simulink model "tqdtqr_rebuild_V3"  (R2021b)
settings: Solver=VariableStepAuto  StartTime=0.0  StopTime=10.0  RelTol=1e-3
undefined symbols (not defined in the file): ATQD_AfterTqMinGain_X_Deg, ATQD_APSCreepBaseTqD_X_kph, ATQD_APSCreepBaseTqD_Y_Deg, ATQD_APSCreepBaseTqR_X_kph, ATQD_APSCreepBaseTqR_Y_Deg, ATQD_APSCreepIterm_X_kph, ATQD_APSCreepIterm_Y_kph, ATQD_APSCreepPterm_X_kph, ATQD_APSCreepPterm_Y_kph, ATQD_APSDecReq_X_kph, ATQD_APSDecReq_Y_mps2, ATQD_APSDecReqCMD_X_kph, ATQD_APSDecReqTs_X_pct, ATQD_APSDecTimeGain_X_Deg, ATQD_APSDecTimeGain_Y_s, ATQD_APSReqLowSpd_X_Deg, ATQD_AutoHoldReleaseBPS_X_Deg, ATQD_AWDLoadTrqnsGain_X_kg, ATQD_AWDLoadTrqnsGain_Y_pct, ATQD_BOSEnBPSPosn_X_kph, ATQD_BOSMap_X_rpm, ATQD_BOSMap_Y_pct, ATQD_CreepBaseTqD_X_kph, ATQD_CreepBaseTqD_Y_Deg, ATQD_CreepBaseTqR_X_kph, ATQD_CreepBaseTqR_Y_Deg, ATQD_CreepBPSDisPosn_X_Deg, ATQD_CreepBPSDisPosnR_X_Deg, ATQD_CreepBPSEnPosn_X_Deg, ATQD_CreepBPSEnPosnR_X_Deg, ATQD_CreepDeltaTq_X_kph, ATQD_CreepIterm_X_kph, ATQD_CreepIterm_Y_kph, ATQD_CreepItermMaxLimit_X_pct, ATQD_CreepPreloadTime_X_kph, ATQD_CreepPreloadTq_X_kph, ATQD_CreepPreloadTq_Y_s, ATQD_CreepProtTq_X_Deg, ATQD_CreepPterm_X_kph, ATQD_CreepPterm_Y_kph, ATQD_CreepRrTqSpRat_X_rpm, ATQD_CreepRrTqSpRat_Y_Nm, ATQD_CreepTargetSpdD_X_pct, ATQD_CreepTargetSpdR_X_pct, ATQD_CreepUpLimitTq_X_rpm, ATQD_DecIneOPDHoldEnDelay_X_Deg, ATQD_DecIneOPDHoldEnDelay_Y_bar, ATQD_ECOTqMapD_X_rpm, ATQD_ECOTqMapD_Y_pct, ATQD_EMTqMapD_X_rpm, ATQD_EMTqMapD_Y_pct, ATQD_EOPDTqMapDCon_X_rpm, ATQD_EOPDTqMapDCon_Y_Deg, ATQD_EstInitVehWeight_X_c, ATQD_FAfterTqCMDGain_X_rpm, ATQD_FAfterTqCMDGain_Y_pct, ATQD_ForceLowSpd_X_Deg, ATQD_ForcePLimitSpd_X_Deg, ATQD_FrLossMAPLowV_X_rpm, ATQD_FrLossMAPLowV_Y_Nm ... (+949)
libraries: simulink x235, hcu_lib x208, tqr x63, tqd x6
(part 30 of 37)

== system tqdtqr_rebuild_V3/Input_Convert/Signal function/SWC1 SWC2 status/SWC2_Subsystem/Speed Setting Mode/ACC Speed Setting ON ==
  note: ACC limit speed setting
  note: ACCSetSpd_241018
  VTQD_SWC2ScrollUpSta_enum : Inport
  VTQD_SWC2ScrollDownSta_enum : Inport  Port=2
  VVMC_LVDAACCStatusInformation_flg : Inport  Port=3
  VTQD_SpdLim4SetSpd_raw32 : Inport  Port=4
  VINP_ADASACCSta_enum : Inport  Port=5
  VINP_Distanceunit_flg : Inport  Port=6
  VINP_SmartEcoModeSW_flg : Inport  Port=7
  VINP_IVIACCAdaptiveSta_flg : Inport  Port=8
  VTQD_Set2MeterSpd_flg : Inport  Port=9
  VTQD_SetRoadSpdLim_flg : Inport  Port=10
  VINP_ADASSLIFSpdLim_enum : Inport  Port=11
  VTQD_LScrollPressShort_flg : Inport  Port=12
  VVMC_MeterIndSpeed_raw32 : Inport  Port=13
  VTQD_SWC2ScrollDownSta_flg : Inport  Port=14
  VTQD_SWC2ScrollUpSta_flg : Inport  Port=15
  VTQD_LastSetSpd_kph : Inport  Port=16
  Action Port : ActionPort  InitializeStates=reset  ActionPortLabel=if(u1 ~= 0)
  " 20" : Constant  Value=KTQD_ACCActiveMetSpdLoMPH_mph
  " 30kph" : Constant  Value=KTQD_ACCActiveMetSpdLo_kph
  105 : Constant  Value=KTQD_ACCActiveMetSpdHiMPH_mph
  180kph : Constant  Value=KTQD_ACCActiveMetSpdHi_kph
  2 : Constant  Value=KTQD_SmartEcoLimitSpd_kph
  3 : Constant  Value=KTQD_SmartEcoLimitSpd_mph
  5 : Constant  Value=KTQD_SetSpdDeltaLongMPH_mph
  5kph : Constant  Value=KTQD_SetSpdDeltaLong_kph
  ACCSetSpd_2506 : Stateflow chart  TreatAsAtomicUnit=on
  AND1 : Logic  AllPortsSameDT=off  OutDataTypeStr=boolean
  Cast To Single : DataTypeConversion  OutDataTypeStr=int8
  Constant126 : Constant  Value=0x0  OutDataTypeStr=uint8
  Equal53 : RelationalOperator  Operator=~=  OutDataTypeStr=boolean  RndMeth=Simplest
  ONE : Constant  Value=ONE_INT
  Relational Operator2 : RelationalOperator  Operator===  OutDataTypeStr=boolean  RndMeth=Simplest
  Relational Operator4 : RelationalOperator  Operator===  OutDataTypeStr=boolean  RndMeth=Simplest
  Round : Rounding  Operator=round
  Switch{1..6} (6 alike) : Switch  Criteria=u2 ~= 0
      settings: AttributesFormatString=%<Criteria>
  standby : Constant  Value=ENUM_ADASACCSTA_STANDBY
  zero : Constant  Value=ZERO_INT
  VTQD_ACCSetSpd_kph : Outport
  wires:
  [VTQD_LastSetSpd_kph] -> ACCSetSpd_2506/18(VTQD_LastSetSpd_kph)
  VTQD_LastSetSpd_kph/1 -> [VTQD_LastSetSpd_kph]
  VTQD_SWC2ScrollUpSta_flg/1 -> [VTQD_SWC2ScrollUpSta_flg]
  VTQD_SWC2ScrollDownSta_flg/1 -> [VTQD_SWC2ScrollDownSta_flg]
  [VTQD_SWC2ScrollDownSta_flg] -> ACCSetSpd_2506/17(VTQD_SWC2ScrollDownSta_flg)
  [VTQD_SWC2ScrollUpSta_flg] -> ACCSetSpd_2506/16(VTQD_SWC2ScrollUpSta_flg)
  [VTQD_ADASSLIFSpdLimDet_flg] -> ACCSetSpd_2506/12(VTQD_ADASSLIFSpdLimDet_flg)
  Equal53/1 -> [VTQD_ADASSLIFSpdLimDet_flg]  "VTQD_ADASSLIFSpdLimDet_flg"
  [VVMC_MeterIndSpeed_raw32] -> ACCSetSpd_2506/15(VVMC_MeterIndSpeed_raw32)
  VVMC_MeterIndSpeed_raw32/1 -> [VVMC_MeterIndSpeed_raw32]
  [VTQD_LScrollPressShort_flg] -> ACCSetSpd_2506/13(VTQD_LScrollPressShort_flg)
  VTQD_LScrollPressShort_flg/1 -> [VTQD_LScrollPressShort_flg]
  [VINP_ADASSLIFSpdLim_enum] -> Equal53/1
  VINP_ADASSLIFSpdLim_enum/1 -> [VINP_ADASSLIFSpdLim_enum]
  [VTQD_SetRoadSpdLim_flg] -> ACCSetSpd_2506/10(VTQD_SetRoadSpdLim_flg)
  VTQD_SetRoadSpdLim_flg/1 -> [VTQD_SetRoadSpdLim_flg]
  [VTQD_Set2MeterSpd_flg] -> ACCSetSpd_2506/6(VTQD_Set2MeterSpd_flg)
  VTQD_Set2MeterSpd_flg/1 -> [VTQD_Set2MeterSpd_flg]
  [VINP_IVIACCAdaptiveSta_flg] -> ACCSetSpd_2506/2(VINP_IVIACCAdaptiveSta_flg)
  VINP_IVIACCAdaptiveSta_flg/1 -> [VINP_IVIACCAdaptiveSta_flg]
  VTQD_SWC2ScrollDownSta_enum/1 -> [VTQD_SWC2ScrollDownSta_enum]
  [VVMC_LVDAACCStatusInformation_flg] -> ACCSetSpd_2506/14(VVMC_LVDAACCStatusInformation_flg)
  [VTQD_ACCSetSpd_raw32] -> Round/1
  ACCSetSpd_2506/1(VTQD_ACCSetSpd_raw32) -> [VTQD_ACCSetSpd_raw32]  "VTQD_ACCSetSpd_raw32"
  Constant126/1 -> Equal53/2
  [VINP_Distanceunit_flg] -> ACCSetSpd_2506/11(VINP_Distanceunit_flg)
  [VTQD_SetSpdDeltaLong_raw32] -> ACCSetSpd_2506/9(VTQD_SetSpdDeltaLong_raw32)
  [VTQD_SWC2ScrollDownSta_enum] -> ACCSetSpd_2506/8(VTQD_SWC2ScrollDownSta_enum)
  [VTQD_SWC2ScrollUpSta_enum] -> ACCSetSpd_2506/7(VTQD_SWC2ScrollUpSta_enum)
  [VTQD_ACCActiveMetSpdLo_raw32] -> ACCSetSpd_2506/5(VTQD_ACCActiveMetSpdLo_raw32)
  [VTQD_ACCActiveMetSpdHi_raw32] -> ACCSetSpd_2506/4(VTQD_ACCActiveMetSpdHi_raw32)
  [VTQD_SpdLim4SetSpd_raw32] -> ACCSetSpd_2506/3(VTQD_SpdLim4SetSpd_raw32)
  [VINP_ADASACCSta_enum] -> ACCSetSpd_2506/1(VINP_ADASACCSta_enum)
  2/1 -> Switch5/1
  3/1 -> Switch6/1
  Switch6/1 -> Switch2/1
  105/1 -> Switch6/3
  [VINP_SmartEcoModeSW_flg] -> Switch6/2
  Switch5/1 -> Switch2/3
  [VINP_SmartEcoModeSW_flg] -> Switch5/2
  180kph/1 -> Switch5/3
  VINP_SmartEcoModeSW_flg/1 -> [VINP_SmartEcoModeSW_flg]
  VTQD_SWC2ScrollUpSta_enum/1 -> [VTQD_SWC2ScrollUpSta_enum]
  Round/1 -> Cast To Single/1
  5/1 -> Switch4/1
  5kph/1 -> Switch4/3
  [VINP_Distanceunit_flg] -> Switch4/2
  " 20"/1 -> Switch3/1
  " 30kph"/1 -> Switch3/3
  [VINP_Distanceunit_flg] -> Switch3/2
  Switch2/1 -> [VTQD_ACCActiveMetSpdHi_raw32]  "VTQD_ACCActiveMetSpdHi_raw32"
  [VINP_Distanceunit_flg] -> Switch2/2
  VINP_Distanceunit_flg/1 -> [VINP_Distanceunit_flg]
  Relational Operator4/1 -> AND1/2
  Relational Operator2/1 -> AND1/1
  zero/1 -> Relational Operator4/2
  standby/1 -> Relational Operator2/2
  ONE/1 -> Switch1/1
  AND1/1 -> Switch1/2
  [VINP_ADASACCSta_enum] -> Relational Operator2/1
  Cast To Single/1 -> Switch1/3, Relational Operator4/1
  VINP_ADASACCSta_enum/1 -> [VINP_ADASACCSta_enum]
  VTQD_SpdLim4SetSpd_raw32/1 -> [VTQD_SpdLim4SetSpd_raw32]
  Switch3/1 -> [VTQD_ACCActiveMetSpdLo_raw32]  "VTQD_ACCActiveMetSpdLo_raw32"
  Switch4/1 -> [VTQD_SetSpdDeltaLong_raw32]  "VTQD_SetSpdDeltaLong_raw32"
  VVMC_LVDAACCStatusInformation_flg/1 -> [VVMC_LVDAACCStatusInformation_flg]
  Switch1/1 -> [VTQD_ACCSetSpd_kph]
  [VTQD_ACCSetSpd_kph] -> VTQD_ACCSetSpd_kph/1

== system tqdtqr_rebuild_V3/Input_Convert/Signal function/SWC1 SWC2 status/SWC2_Subsystem/Speed Setting Mode/CC Speed Setting ON ==
  note: CC speed calculate
  note: CC limit speed setting
  VVMC_CCCtrlSta_enum : Inport
  "VTQD_SWCResUpPress_enum  " : Inport  Port=2
  "VTQD_SWCSetDownPress_enum  " : Inport  Port=3
  VTQD_SpdLim4SetSpd_raw32 : Inport  Port=4
  VTQD_SetSpdDeltaLongFit_kph : Inport  Port=5
  VINP_Distanceunit_flg : Inport  Port=6
  VINP_SmartEcoModeSW_flg : Inport  Port=7
  Action Port : ActionPort  InitializeStates=reset  ActionPortLabel=elseif(u2 ~= 0)
  " 1" : Constant  Value=KTQD_CCActiveMetSpdLo_kph
  " 2" : Constant  Value=KTQD_CCActiveMetSpdLoMPH_mph
  1 : Constant  Value=KTQD_SetSpdDeltaLongFit_kph
  2 : Constant  Value=KTQD_SetSpdDeltaShort_kph
  3 : Constant  Value=KTQD_CCActiveMetSpdHi_kph
  4 : Constant  Value=KTQD_SetSpdDeltaLong_kph
  5 : Constant  Value=KTQD_CCActiveMetSpdHiMPH_mph
  6 : Constant  Value=KTQD_SetSpdDeltaLongMPH_mph
  7 : Constant  Value=KTQD_SmartEcoLimitSpd_kph
  8 : Constant  Value=KTQD_SmartEcoLimitSpd_mph
  AND1 : Logic  AllPortsSameDT=off  OutDataTypeStr=boolean
  CC Speed Setting Mode : Stateflow chart  TreatAsAtomicUnit=on
      settings: PortSchema="{\"entries\":[{\"content\":{\"sides\":[{\"content\":{\"connectorIds\":[\"In5\",\"In12\",\"In4\",\"In3\",\"In9\",\"In6\",\"In7\",\"In8\",\"In1\",\"In2\",\"In11\",\"In10\"]},\"type\":\"ConnectorPlacement.EquallySpacedRectSide\",\"uuid\":\"331c8dfa-4564-419d-9323-fdbf8561d50b\"},{\"content\":{\"connectorIds\":[\"Out1\",\"Out2\"],\"side\":\"RIGHT\"},\"type\":\"ConnectorPlacement.EquallySpacedRectSide\",\"uuid\":\"71cb1444-7708-4b6f-91dd-d8a1c8c14ea8\"},{\"content\":{\"connectorIds\":[],\"side\":\"TOP\"},\"type\":\"ConnectorPlacement.EquallySpacedRectSide\",\"uuid\":\"6ecf38bb-d171-491a-a8b2-073f135e7039\"}]},\"type\":\"ConnectorPlacement.EquallySpacedConnector\",\"uuid\":\"fc3afa97-6e6e-4933-9aff-7c8f8cbb1702\"}],\"packageUris\":[\"http://schema.mathworks.com/mf0/Connector/R2020b\"],\"version\":\"1.0\"}"
  Cast To Single : DataTypeConversion  OutDataTypeStr=int8
  ONE : Constant  Value=ONE_INT
  Relational Operator2 : RelationalOperator  Operator===  OutDataTypeStr=boolean  RndMeth=Simplest
  Relational Operator4 : RelationalOperator  Operator===  OutDataTypeStr=boolean  RndMeth=Simplest
  Round : Rounding  Operator=round
  Specific_STATE_ChangeToSTANDBY : Stateflow chart  TreatAsAtomicUnit=on
  Switch{1,3..6} (5 alike) : Switch  Criteria=u2 ~= 0
      settings: AttributesFormatString=%<Criteria>
  Switch2 : Switch  Criteria=u2 > Threshold
  Terminator : Terminator
  standby : Constant  Value=ENUM_ADASCCSTA_STANDBY
  zero : Constant  Value=ZERO_INT
  VTQD_CCSetSpd_kph : Outport
  wires:
  7/1 -> Switch6/1
  8/1 -> Switch5/1
  Switch5/1 -> Switch2/1
  [VINP_SmartEcoModeSW_flg] -> Switch5/2
  5/1 -> Switch5/3
  Switch6/1 -> Switch2/3
  3/1 -> Switch6/3
  [VINP_SmartEcoModeSW_flg] -> Switch6/2
  VINP_SmartEcoModeSW_flg/1 -> [VINP_SmartEcoModeSW_flg]
  CC Speed Setting Mode/1(VTQD_CCSetSpd_kph) -> Round/1
  Round/1 -> Cast To Single/1
  [VINP_Distanceunit_flg] -> CC Speed Setting Mode/6(VINP_Distanceunit_flg)
  6/1 -> Switch4/1
  4/1 -> Switch4/3
  [VINP_Distanceunit_flg] -> Switch4/2
  " 2"/1 -> Switch3/1
  " 1"/1 -> Switch3/3
  [VINP_Distanceunit_flg] -> Switch3/2
  VINP_Distanceunit_flg/1 -> [VINP_Distanceunit_flg]
  [VINP_Distanceunit_flg] -> Switch2/2
  Relational Operator4/1 -> AND1/2
  Relational Operator2/1 -> AND1/1
  zero/1 -> Relational Operator4/2
  standby/1 -> Relational Operator2/2
  ONE/1 -> Switch1/1
  AND1/1 -> Switch1/2
  [VVMC_CCCtrlSta_enum] -> Relational Operator2/1
  Cast To Single/1 -> Switch1/3, Relational Operator4/1
  1/1 -> CC Speed Setting Mode/3(KTQD_SetSpdDeltaLongFit_kph)
  2/1 -> CC Speed Setting Mode/2(KTQD_SetSpdDeltaShort_kph)
  VVMC_CCCtrlSta_enum/1 -> [VVMC_CCCtrlSta_enum]
  [VVMC_CCCtrlSta_enum] -> Specific_STATE_ChangeToSTANDBY/1(VVMC_CCCtrlSta_enum)
  Specific_STATE_ChangeToSTANDBY/1(VTQD_CCChangeToSTANDBY_flg) -> [VTQD_ChangeToSTANDBY_flg]
  [VTQD_ChangeToSTANDBY_flg] -> CC Speed Setting Mode/12(VTQD_ChangeToSTANDBY_flg)
  CC Speed Setting Mode/2(VTQD_CCSpdResetFinish_flg) -> Terminator/1
  [VVMC_CCCtrlSta_enum] -> CC Speed Setting Mode/5(VVMC_CCCtrlSta_enum)
  "VTQD_SWCResUpPress_enum  "/1 -> [VTQD_SWCResUpPress_enum]
  [VTQD_SWCResUpPress_enum] -> CC Speed Setting Mode/11(VTQD_SWCResUpPress_enum)
  "VTQD_SWCSetDownPress_enum  "/1 -> [VTQD_SWCSetDownPress_enum]
  [VTQD_SWCSetDownPress_enum] -> CC Speed Setting Mode/10(VTQD_SWCSetDownPress_enum)
  VTQD_SpdLim4SetSpd_raw32/1 -> [VTQD_SpdLim4SetSpd_raw32]
  [VTQD_SpdLim4SetSpd_raw32] -> CC Speed Setting Mode/9(VVMC_MeterIndSpeed_raw32)
  VTQD_SetSpdDeltaLongFit_kph/1 -> [VTQD_SetSpdDeltaLongFit_kph]
  [VTQD_SetSpdDeltaLongFit_kph] -> CC Speed Setting Mode/4(VTQD_SetSpdDeltaLongFit_kph)
  Switch2/1 -> [KTQD_CCActiveMetSpdHi_raw32]
  [KTQD_CCActiveMetSpdHi_raw32] -> CC Speed Setting Mode/7(KTQD_CCActiveMetSpdHi_raw32)
  Switch3/1 -> [KTQD_CCActiveMetSpdLo_raw32]
  [KTQD_CCActiveMetSpdLo_raw32] -> CC Speed Setting Mode/8(KTQD_CCActiveMetSpdLo_raw32)
  Switch4/1 -> [KTQD_SetSpdDeltaLong_kph]
  [KTQD_SetSpdDeltaLong_kph] -> CC Speed Setting Mode/1(KTQD_SetSpdDeltaLong_kph)
  Switch1/1 -> [VTQD_CCSetSpd_kph]
  [VTQD_CCSetSpd_kph] -> VTQD_CCSetSpd_kph/1

== system tqdtqr_rebuild_V3/Input_Convert/Signal function/SWC1 SWC2 status/SWC2_Subsystem/Speed Setting Mode/Else Speed Setting On ==
  In : Inport
  Action Port : ActionPort  ActionPortLabel=else
  Data Type Conversion : DataTypeConversion
  Out : Outport
  wires:
  In/1 -> Data Type Conversion/1
  Data Type Conversion/1 -> Out/1

== system tqdtqr_rebuild_V3/Input_Convert/Signal function/SWC1 SWC2 status/SWC2_Subsystem/Speed Setting Mode/ISA Speed Setting ON ==
  VINP_ADASSLIFSpdLim_enum : Inport
  VINP_SmartEcoModeSW_flg : Inport  Port=2
  Action Port : ActionPort  ActionPortLabel=elseif( u4~= 0)
  8 : Constant  Value=KTQD_SmartEcoLimitSpd_kph
  Data Type Conversion : DataTypeConversion
  Min : MinMax  Inputs=2
  Switch : Switch  Criteria=u2 > Threshold
  VTQD_ISASetSpd_kph : Outport
  wires:
  Switch/1 -> Data Type Conversion/1
  8/1 -> Min/1
  Min/1 -> Switch/1
  VINP_ADASSLIFSpdLim_enum/1 -> Switch/3, Min/2
  VINP_SmartEcoModeSW_flg/1 -> Switch/2
  Data Type Conversion/1 -> VTQD_ISASetSpd_kph/1

== system tqdtqr_rebuild_V3/Input_Convert/Signal function/SWC1 SWC2 status/SWC2_Subsystem/Speed Setting Mode/MSA Speed Setting ON ==
  note: Calulate MSA speed and ouput
  note: MSA limit speed setting
  VVMC_MSACrlSta_enum : Inport
  "VTQD_SWC2ScrollUpSta_enum  " : Inport  Port=2
  "VTQD_SWC2ScrollDownSta_enum  " : Inport  Port=3
  VTQD_SpdLim4SetSpd_raw32 : Inport  Port=4
  VINP_Distanceunit_flg : Inport  Port=5
  VINP_SmartEcoModeSW_flg : Inport  Port=6
  VINP_IVIACCAdaptiveSta_flg : Inport  Port=7
  VTQD_Set2MeterSpd_flg : Inport  Port=8
  VTQD_SetRoadSpdLim_flg : Inport  Port=9
  VINP_ADASSLIFSpdLim_enum : Inport  Port=10
  VTQD_LScrollPressShort_flg : Inport  Port=11
  VVMC_MeterIndSpeed_raw32 : Inport  Port=12
  VTQD_LastSetSpd_kph : Inport  Port=13
  Action Port : ActionPort  InitializeStates=reset  ActionPortLabel=elseif( u3~= 0)
  " 1" : Constant  Value=KTQD_MSAActiveMetSpdLoMPH_mph
  " 80" : Constant  Value=KTQD_MSAActiveMetSpdLo_kph
  160 : Constant  Value=KTQD_MSAActiveMetSpdHi_kph
  2 : Constant  Value=KTQD_MSAActiveMetSpdHiMPH_mph
  3 : Constant  Value=KTQD_SetSpdDeltaLongMPH_mph
  4 : Constant  Value=KTQD_SmartEcoLimitSpd_mph
  5 : Constant  Value=KTQD_SetSpdDeltaLong_kph
  6 : Constant  Value=KTQD_SmartEcoLimitSpd_kph
  AND : Logic  AllPortsSameDT=off  OutDataTypeStr=boolean
  AND1 : Logic  AllPortsSameDT=off  OutDataTypeStr=boolean
  Cast To Single : DataTypeConversion  OutDataTypeStr=int8
  Constant126 : Constant  Value=0x0  OutDataTypeStr=uint8
  Equal53 : RelationalOperator  Operator=~=  OutDataTypeStr=boolean  RndMeth=Simplest
  KTQD_ISATestSW_flg : Constant  Value=KTQD_ISATestSW_flg
  MSASetSpd_241018 : Stateflow chart  AncestorBlock=tqd/TQD/TorqueDemand/Signal_convert/SWC2_Subsystem/Speed Setting Mode/MSA Speed Setting ON/MSASetSpd_241018  TreatAsAtomicUnit=on
  ONE : Constant  Value=ONE_INT
  Relational Operator2 : RelationalOperator  Operator===  OutDataTypeStr=boolean  RndMeth=Simplest
  Relational Operator4 : RelationalOperator  Operator===  OutDataTypeStr=boolean  RndMeth=Simplest
  Round : Rounding  Operator=round
  Switch{1..6} (6 alike) : Switch  Criteria=u2 ~= 0
      settings: AttributesFormatString=%<Criteria>
  standby : Constant  Value=ENUM_ADASMSASTA_STANDBY
  zero : Constant  Value=ZERO_INT
  VSCP_MSASetSpd_kph : Outport
  wires:
  [VTQD_LastSetSpd_kph] -> MSASetSpd_241018/15(VTQD_LastSetSpd_kph)
  VTQD_LastSetSpd_kph/1 -> [VTQD_LastSetSpd_kph]
  Equal53/1 -> MSASetSpd_241018/12(VTQD_ADASSLIFSpdLimDet_flg)
  Constant126/1 -> Equal53/2
  [VINP_ADASSLIFSpdLim_enum] -> Equal53/1
  [VTQD_SetSpdDeltaLong_kph] -> MSASetSpd_241018/9(VTQD_SetSpdDeltaLong_raw32)
  [VVMC_MeterIndSpeed_raw32] -> MSASetSpd_241018/14(VVMC_MeterIndSpeed_raw32)
  VVMC_MeterIndSpeed_raw32/1 -> [VVMC_MeterIndSpeed_raw32]
  [VTQD_LScrollPressShort_flg] -> MSASetSpd_241018/13(VTQD_LScrollPressShort_flg)
  VTQD_LScrollPressShort_flg/1 -> [VTQD_LScrollPressShort_flg]
  VINP_ADASSLIFSpdLim_enum/1 -> [VINP_ADASSLIFSpdLim_enum]
  [VTQD_SetRoadSpdLim_flg] -> MSASetSpd_241018/10(VTQD_SetRoadSpdLim_flg)
  VTQD_SetRoadSpdLim_flg/1 -> [VTQD_SetRoadSpdLim_flg]
  [VTQD_Set2MeterSpd_flg] -> MSASetSpd_241018/6(VTQD_Set2MeterSpd_flg)
  VTQD_Set2MeterSpd_flg/1 -> [VTQD_Set2MeterSpd_flg]
  [VINP_IVIACCAdaptiveSta_flg] -> AND/1
  VINP_IVIACCAdaptiveSta_flg/1 -> [VINP_IVIACCAdaptiveSta_flg]
  Switch4/1 -> [VTQD_SetSpdDeltaLong_kph]  "VTQD_SetSpdDeltaLong_kph"
  [VTQD_MSASetSpd_raw32] -> Round/1
  MSASetSpd_241018/1(VTQD_MSASetSpd_raw32) -> [VTQD_MSASetSpd_raw32]  "VTQD_MSASetSpd_raw32"
  [VINP_Distanceunit_flg] -> MSASetSpd_241018/11(VINP_Distanceunit_flg)
  [VTQD_SWC2ScrollDownSta_enum] -> MSASetSpd_241018/8(VTQD_SWC2ScrollDownSta_enum)
  [VTQD_SWC2ScrollUpSta_enum] -> MSASetSpd_241018/7(VTQD_SWC2ScrollUpSta_enum)
  [VTQD_MSAActiveMetSpdLo_raw32] -> MSASetSpd_241018/5(VTQD_MSAActiveMetSpdLo_raw32)
  [VTQD_MSAActiveMetSpdHi_raw32] -> MSASetSpd_241018/4(VTQD_MSAActiveMetSpdHi_raw32)
  [VTQD_SpdLim4SetSpd_raw32] -> MSASetSpd_241018/3(VTQD_SpdLim4SetSpd_raw32)
  KTQD_ISATestSW_flg/1 -> AND/2
  AND/1 -> MSASetSpd_241018/2(VINP_IVIACCAdaptiveSta_flg)
  [VVMC_MSACrlSta_enum] -> MSASetSpd_241018/1(VVMC_MSACrlSta_enum)
  6/1 -> Switch6/1
  4/1 -> Switch5/1
  Switch5/1 -> Switch2/1
  2/1 -> Switch5/3
  [VINP_SmartEcoModeSW_flg] -> Switch5/2
  Switch6/1 -> Switch2/3
  160/1 -> Switch6/3
  [VINP_SmartEcoModeSW_flg] -> Switch6/2
  VINP_SmartEcoModeSW_flg/1 -> [VINP_SmartEcoModeSW_flg]
  Round/1 -> Cast To Single/1
  3/1 -> Switch4/1
  5/1 -> Switch4/3
  [VINP_Distanceunit_flg] -> Switch4/2
  " 1"/1 -> Switch3/1
  " 80"/1 -> Switch3/3
  [VINP_Distanceunit_flg] -> Switch3/2
  VINP_Distanceunit_flg/1 -> [VINP_Distanceunit_flg]
  [VINP_Distanceunit_flg] -> Switch2/2
  Relational Operator4/1 -> AND1/2
  [VVMC_MSACrlSta_enum] -> Relational Operator2/1
  Relational Operator2/1 -> AND1/1
  Cast To Single/1 -> Switch1/3, Relational Operator4/1
  ONE/1 -> Switch1/1
  standby/1 -> Relational Operator2/2
  zero/1 -> Relational Operator4/2
  AND1/1 -> Switch1/2
  "VTQD_SWC2ScrollUpSta_enum  "/1 -> [VTQD_SWC2ScrollUpSta_enum]
  "VTQD_SWC2ScrollDownSta_enum  "/1 -> [VTQD_SWC2ScrollDownSta_enum]
  VVMC_MSACrlSta_enum/1 -> [VVMC_MSACrlSta_enum]
  Switch3/1 -> [VTQD_MSAActiveMetSpdLo_raw32]  "VTQD_MSAActiveMetSpdLo_raw32"
  Switch2/1 -> [VTQD_MSAActiveMetSpdHi_raw32]  "VTQD_MSAActiveMetSpdHi_raw32"
  VTQD_SpdLim4SetSpd_raw32/1 -> [VTQD_SpdLim4SetSpd_raw32]
  Switch1/1 -> [VSCP_MSASetSpd_kph]
  [VSCP_MSASetSpd_kph] -> VSCP_MSASetSpd_kph/1

== system tqdtqr_rebuild_V3/Input_Convert/Signal function/SWC1 SWC2 status/SWC2_Subsystem/Speed Setting Mode/SWC2ScrollDownSta ==
  note: Long press or Short press
  INPUT : Inport
  task_time_s : Inport  Port=2
  AND : Logic  AllPortsSameDT=off  OutDataTypeStr=boolean
  AND1 : Logic  AllPortsSameDT=off  OutDataTypeStr=boolean
  Constant1 : Constant  Value=ENUM_SWCBOTTONPRESS_LONGPRESS
  Constant2 : Constant  Value=KTQD_ScrollDownShortPLim_s
  Constant3 : Constant  Value=KTQD_ScrollDownLongPLim_s
  Constant7 : Constant  Value=ENUM_SWCBOTTONPRESS_SHORTPRESS
  Constant8 : Constant  Value=ENUM_SWCBOTTONPRESS_NOPRESS
  Delay : Delay  DelayLength=1  InitialCondition=boolean(0)
  DelayEnable_LONG_PRESS1 : hcu_lib/Basic_Blocks/DelayEnable
  DelayEnable_SHORT_PRESS1 : hcu_lib/Basic_Blocks/DelayEnable
  Detect Decrease : simulink/Logic and Bit Operations/Detect Decrease  vinit=boolean(0)  OutDataTypeStr=boolean
  Detect Decrease4 : simulink/Logic and Bit Operations/Detect Decrease  vinit=boolean(0)  OutDataTypeStr=boolean
  NOT : Logic  Operator=NOT  AllPortsSameDT=off  OutDataTypeStr=boolean
  NOT1 : Logic  Operator=NOT  AllPortsSameDT=off  OutDataTypeStr=boolean
  SR_Latch : hcu_lib/Basic_Blocks/SR_Latch
  Switch : Switch  Criteria=u2 ~= 0
      settings: AttributesFormatString=%<Criteria>
  Switch3 : Switch  Criteria=u2 ~= 0
      settings: AttributesFormatString=%<Criteria>
  OUTPUT : Outport
  wires:
  Switch/1 -> OUTPUT/1
  Constant8/1 -> Switch3/3
  Constant1/1 -> Switch/1
  Constant7/1 -> Switch3/1
  [Long_press_falling_edge] -> Switch/2
  Detect Decrease4/1 -> [Short_press_falling_Edge]
  [task_time_s] -> DelayEnable_LONG_PRESS1/3
  [task_time_s] -> DelayEnable_SHORT_PRESS1/3
  Constant2/1 -> DelayEnable_SHORT_PRESS1/2
  Constant3/1 -> DelayEnable_LONG_PRESS1/2
  DelayEnable_SHORT_PRESS1/1 -> Detect Decrease4/1
  Switch3/1 -> Switch/3
  DelayEnable_LONG_PRESS1/1 -> [Long_press_falling_edge]
  task_time_s/1 -> [task_time_s]
  INPUT/1 -> [INPUT]
  [Long_press_falling_edge] -> Delay/1
  Delay/1 -> NOT/1
  NOT/1 -> AND/2
  AND/1 -> DelayEnable_LONG_PRESS1/1
  [INPUT] -> AND/1
  [Long_press_falling_edge] -> SR_Latch/1
  AND1/1 -> DelayEnable_SHORT_PRESS1/1
  [INPUT] -> AND1/1
  SR_Latch/1 -> NOT1/1
  NOT1/1 -> AND1/2
  [INPUT] -> Detect Decrease/1
  Detect Decrease/1 -> SR_Latch/2
  [Short_press_falling_Edge] -> Switch3/2

== system tqdtqr_rebuild_V3/Input_Convert/Signal function/SWC1 SWC2 status/SWC2_Subsystem/Speed Setting Mode/SWC2ScrollUpSta ==
  note: Long press or Short press
  INPUT : Inport
  task_time_s : Inport  Port=2
  AND : Logic  AllPortsSameDT=off  OutDataTypeStr=boolean
  AND1 : Logic  AllPortsSameDT=off  OutDataTypeStr=boolean
  Constant2 : Constant  Value=KTQD_ScrollUpShortPLim_s
  Constant3 : Constant  Value=KTQD_ScrollUpLongPLim_s
  Constant4 : Constant  Value=ENUM_SWCBOTTONPRESS_LONGPRESS
  Constant5 : Constant  Value=ENUM_SWCBOTTONPRESS_SHORTPRESS
  Constant6 : Constant  Value=ENUM_SWCBOTTONPRESS_NOPRESS
  Delay : Delay  DelayLength=1  InitialCondition=boolean(0)
      settings: AttributesFormatString=%<InitialCondition>
  DelayEnable_LONG_PRESS1 : hcu_lib/Basic_Blocks/DelayEnable
  DelayEnable_SHORT_PRESS1 : hcu_lib/Basic_Blocks/DelayEnable
  Detect Decrease : simulink/Logic and Bit Operations/Detect Decrease  vinit=boolean(0)  OutDataTypeStr=boolean
  Detect Decrease4 : simulink/Logic and Bit Operations/Detect Decrease  vinit=boolean(0)  OutDataTypeStr=boolean
  NOT : Logic  Operator=NOT  AllPortsSameDT=off  OutDataTypeStr=boolean
  NOT1 : Logic  Operator=NOT  AllPortsSameDT=off  OutDataTypeStr=boolean
  SR_Latch : hcu_lib/Basic_Blocks/SR_Latch
  Switch : Switch  Criteria=u2 ~= 0
      settings: AttributesFormatString=%<Criteria>
  Switch3 : Switch  Criteria=u2 ~= 0
      settings: AttributesFormatString=%<Criteria>
  OUTPUT : Outport
  wires:
  Switch/1 -> OUTPUT/1
  Constant6/1 -> Switch3/3
  Constant4/1 -> Switch/1
  Constant5/1 -> Switch3/1
  [Long_press_falling_edge] -> Switch/2
  Detect Decrease4/1 -> [Short_press_falling_Edge]
  [task_time_s] -> DelayEnable_LONG_PRESS1/3
  [task_time_s] -> DelayEnable_SHORT_PRESS1/3
  Constant2/1 -> DelayEnable_SHORT_PRESS1/2
  Constant3/1 -> DelayEnable_LONG_PRESS1/2
  DelayEnable_SHORT_PRESS1/1 -> Detect Decrease4/1
  Switch3/1 -> Switch/3
  DelayEnable_LONG_PRESS1/1 -> [Long_press_falling_edge]
  task_time_s/1 -> [task_time_s]
  INPUT/1 -> [INPUT]
  [Long_press_falling_edge] -> Delay/1
  Delay/1 -> NOT/1
  NOT/1 -> AND/2
  AND/1 -> DelayEnable_LONG_PRESS1/1
  [INPUT] -> AND/1
  [Long_press_falling_edge] -> SR_Latch/1
  AND1/1 -> DelayEnable_SHORT_PRESS1/1
  [INPUT] -> AND1/1
  SR_Latch/1 -> NOT1/1
  NOT1/1 -> AND1/2
  [INPUT] -> Detect Decrease/1
  Detect Decrease/1 -> SR_Latch/2
  [Short_press_falling_Edge] -> Switch3/2

== system tqdtqr_rebuild_V3/Input_Convert/Signal function/SWC1 SWC2 status/SWC_Subsystem/Speed Setting Mode/ACC Speed Setting ON ==
  note: Allow to set speed
  note: ACC SPEED SETTING MODE
  VTQD_SWCResUpSta_flg : Inport
  VTQD_SWCSetDownSta_flg : Inport  Port=2
  task_time_s : Inport  Port=3
  VVMC_LVDAACCStatusInformation_flg : Inport  Port=4
  VVMC_ACCObjDist_m : Inport  Port=5
  VVMC_MeterIndSpeed_raw32 : Inport  Port=6
  VINP_ADASACCSta_enum : Inport  Port=7
  VINP_Distanceunit_flg : Inport  Port=8
  VINP_SmartEcoModeSW_flg : Inport  Port=9
  VVMC_SetACCDisableAPS_flg : Inport  Port=10
  Action Port : ActionPort  InitializeStates=reset  ActionPortLabel=if(u1 ~= 0)
  " 20" : Constant  Value=KTQD_ACCActiveMetSpdLoMPH_mph
  " 30kph" : Constant  Value=KTQD_ACCActiveMetSpdLo_kph
  0 : Constant  Value=KTQD_AllowSetSpdOvrd_flg
  1 : Constant  Value=KTQD_AllowSetSpdOvrdVal_flg
  1.1s : Constant  Value=KTQD_SetSpdLongPLim_s
  105 : Constant  Value=KTQD_ACCActiveMetSpdHiMPH_mph
  10kph1 : Constant  Value=KTQD_AllowSetSpdSpd_kph
  180kph : Constant  Value=KTQD_ACCActiveMetSpdHi_kph
  2 : Constant  Value=KTQD_SmartEcoLimitSpd_kph
  20m : Constant  Value=KVMC_AllowSetSpdDist_m
  2m : Constant  Value=KVMC_NotAllowSetSpdDist_m
  3 : Constant  Value=KTQD_SmartEcoLimitSpd_kph
  5 : Constant  Value=KTQD_SetSpdDeltaLongMPH_mph
  5kph : Constant  Value=KTQD_SetSpdDeltaLong_kph
  ACCSetSpd_Chart_W : Stateflow chart  TreatAsAtomicUnit=on
      settings: PortSchema="{\"entries\":[{\"content\":{\"sides\":[{\"content\":{\"connectorIds\":[\"In1\",\"In2\",\"In3\",\"In4\",\"In5\",\"In6\",\"In7\",\"In8\",\"In12\",\"In9\",\"In10\",\"In11\"]},\"type\":\"ConnectorPlacement.EquallySpacedRectSide\",\"uuid\":\"61ce72b2-2f56-4065-9e06-1345412a8c86\"},{\"content\":{\"connectorIds\":[\"Out1\"],\"side\":\"RIGHT\"},\"type\":\"ConnectorPlacement.EquallySpacedRectSide\",\"uuid\":\"4594d6d3-f7cd-4711-8df0-9a0a2c5601b5\"},{\"content\":{\"connectorIds\":[],\"side\":\"TOP\"},\"type\":\"ConnectorPlacement.EquallySpacedRectSide\",\"uuid\":\"a8857ab2-f9b0-4737-b2f3-522f42c1ada3\"}]},\"type\":\"ConnectorPlacement.EquallySpacedConnector\",\"uuid\":\"0a7f8e6a-9c19-454d-bd26-d3d8923cc49e\"}],\"packageUris\":[\"http://schema.mathworks.com/mf0/Connector/R2020b\"],\"version\":\"1.0\"}"
  AND : Logic  AllPortsSameDT=off  OutDataTypeStr=boolean
  AND1 : Logic  AllPortsSameDT=off  OutDataTypeStr=boolean
  Cast To Single : DataTypeConversion  OutDataTypeStr=int8
  Data Type Conversion : DataTypeConversion  OutDataTypeStr=uint8
  Data Type Conversion1 : DataTypeConversion  OutDataTypeStr=uint8
  Logical Operator : Logic  AllPortsSameDT=off  OutDataTypeStr=boolean
  ONE : Constant  Value=ONE_INT
  OR : Logic  Operator=OR  AllPortsSameDT=off  OutDataTypeStr=boolean
  Product : Product
  Relational Operator : RelationalOperator  Operator=<=  OutDataTypeStr=boolean  RndMeth=Simplest
  Relational Operator1 : RelationalOperator  Operator=>  OutDataTypeStr=boolean  RndMeth=Simplest
  Relational Operator2 : RelationalOperator  Operator===  OutDataTypeStr=boolean  RndMeth=Simplest
  Relational Operator3 : RelationalOperator  OutDataTypeStr=boolean  RndMeth=Simplest
  Relational Operator4 : RelationalOperator  Operator===  OutDataTypeStr=boolean  RndMeth=Simplest
  Round : Rounding  Operator=round
  Switch{,1..6} (7 alike) : Switch  Criteria=u2 ~= 0
      settings: AttributesFormatString=%<Criteria>
  standby : Constant  Value=ENUM_ADASACCSTA_STANDBY
  zero : Constant  Value=ZERO_INT
  zero1 : Constant  Value=KPH2MPH
  VTQD_ACCSetSpd_kph : Outport
  wires:
  Logical Operator/1 -> Switch/3
  OR/1 -> Logical Operator/1
  Data Type Conversion1/1 -> Switch5/1
  Data Type Conversion/1 -> Switch6/1
  [VINP_SmartEcoModeSW_flg] -> Switch5/2
  [VINP_SmartEcoModeSW_flg] -> Switch6/2
  [VINP_Distanceunit_flg] -> Switch2/2
  3/1 -> Data Type Conversion1/1
  Switch6/1 -> Switch2/1
  Switch5/1 -> Switch2/3
  105/1 -> Switch6/3
  Product/1 -> Data Type Conversion/1
  zero1/1 -> Product/2
  2/1 -> Product/1
  180kph/1 -> Switch5/3
  VINP_SmartEcoModeSW_flg/1 -> [VINP_SmartEcoModeSW_flg]
  Round/1 -> Cast To Single/1
  [VINP_Distanceunit_flg] -> ACCSetSpd_Chart_W/6(VINP_Distanceunit_flg)
  5/1 -> Switch4/1
  5kph/1 -> Switch4/3
  [VINP_Distanceunit_flg] -> Switch4/2
  " 20"/1 -> Switch3/1
  " 30kph"/1 -> Switch3/3
  [VINP_Distanceunit_flg] -> Switch3/2
  VINP_Distanceunit_flg/1 -> [VINP_Distanceunit_flg]
  Relational Operator4/1 -> AND1/2
  Relational Operator2/1 -> AND1/1
  zero/1 -> Relational Operator4/2
  standby/1 -> Relational Operator2/2
  ONE/1 -> Switch1/1
  AND1/1 -> Switch1/2
  [VINP_ADASACCSta_enum] -> Relational Operator2/1
  Cast To Single/1 -> Switch1/3, Relational Operator4/1
  [VTQD_AllowSetSpd_flg] -> ACCSetSpd_Chart_W/11(VTQD_AllowSetSpd_flg)
  1/1 -> Switch/1
  0/1 -> Switch/2
  Switch/1 -> [VTQD_AllowSetSpd_flg]  "VTQD_SWCAllowSetSpd_flg"
  Relational Operator3/1 -> OR/2
  AND/1 -> OR/1
  10kph1/1 -> Relational Operator3/2
  [VVMC_MeterIndSpeed_raw32] -> Relational Operator3/1
  Relational Operator1/1 -> AND/2
  Relational Operator/1 -> AND/1
  2m/1 -> Relational Operator1/2
  20m/1 -> Relational Operator/2
  1.1s/1 -> ACCSetSpd_Chart_W/9(KTQD_SetSpdLongPLim_s)
  VTQD_SWCResUpSta_flg/1 -> [VTQD_SWCResUpSta_flg]
  [VTQD_SWCResUpSta_flg] -> ACCSetSpd_Chart_W/2(VTQD_SWCResUpSta_flg)
  VINP_ADASACCSta_enum/1 -> [VINP_ADASACCSta_enum]
  [VINP_ADASACCSta_enum] -> ACCSetSpd_Chart_W/1(VINP_ADASACCSta_enum)
  VTQD_SWCSetDownSta_flg/1 -> [VTQD_SWCSetDownSta_flg]
  [VTQD_SWCSetDownSta_flg] -> ACCSetSpd_Chart_W/3(VTQD_SWCSetDownSta_flg)
  VVMC_MeterIndSpeed_raw32/1 -> [VVMC_MeterIndSpeed_raw32]
  [VVMC_MeterIndSpeed_raw32] -> ACCSetSpd_Chart_W/4(VVMC_MeterIndSpeed_raw32)
  task_time_s/1 -> [task_time_s]
  [task_time_s] -> ACCSetSpd_Chart_W/12(task_time_s)
  VVMC_LVDAACCStatusInformation_flg/1 -> [VVMC_LVDAACCStatusInformation_flg]
  [VVMC_LVDAACCStatusInformation_flg] -> ACCSetSpd_Chart_W/10(VVMC_LVDAACCStatusInformation_flg)
  [KTQD_ACCActiveMetSpdLo_raw32] -> ACCSetSpd_Chart_W/7(KTQD_ACCActiveMetSpdLo_raw32)
  Switch3/1 -> [KTQD_ACCActiveMetSpdLo_raw32]
  [KTQD_SetSpdDeltaLong_kph] -> ACCSetSpd_Chart_W/8(KTQD_SetSpdDeltaLong_kph)
  Switch4/1 -> [KTQD_SetSpdDeltaLong_kph]
  Switch2/1 -> [KTQD_ACCActiveMetSpdHi_raw32]
  [KTQD_ACCActiveMetSpdHi_raw32] -> ACCSetSpd_Chart_W/5(KTQD_ACCActiveMetSpdHi_raw32)
  Switch1/1 -> [VTQD_ACCSetSpd_kph]
  ACCSetSpd_Chart_W/1(VTQD_ACCSetSpd_kph) -> Round/1
  [VTQD_ACCSetSpd_kph] -> VTQD_ACCSetSpd_kph/1
  VVMC_ACCObjDist_m/1 -> [VVMC_ACCObjDist_m]
  [VVMC_ACCObjDist_m] -> Relational Operator/1
  [VVMC_ACCObjDist_m] -> Relational Operator1/1
  [VVMC_SetACCDisableAPS_flg] -> Logical Operator/2
  VVMC_SetACCDisableAPS_flg/1 -> [VVMC_SetACCDisableAPS_flg]

== system tqdtqr_rebuild_V3/Input_Convert/Signal function/SWC1 SWC2 status/SWC_Subsystem/Speed Setting Mode/CC Speed Setting ON ==
  note: CC SPEED SETTING MODE
  VVMC_CCCtrlSta_enum : Inport
  "VTQD_SWCResUpPress_enum  " : Inport  Port=2
  "VTQD_SWCSetDownPress_enum  " : Inport  Port=3
  VVMC_MeterIndSpeed_raw32 : Inport  Port=4
  VTQD_SetSpdDeltaLongFit_kph : Inport  Port=5
  VINP_Distanceunit_flg : Inport  Port=6
  VINP_SmartEcoModeSW_flg : Inport  Port=7
  Action Port : ActionPort  InitializeStates=reset  ActionPortLabel=elseif(u2 ~= 0)
  " 1" : Constant  Value=KTQD_CCActiveMetSpdLo_kph
  " 2" : Constant  Value=KTQD_CCActiveMetSpdLoMPH_mph
  1 : Constant  Value=KTQD_SetSpdDeltaLongFit_kph
  2 : Constant  Value=KTQD_SetSpdDeltaShort_kph
  3 : Constant  Value=KTQD_SmartEcoLimitSpd_kph
  4 : Constant  Value=KTQD_SetSpdDeltaLong_kph
  5 : Constant  Value=KTQD_SmartEcoLimitSpd_kph
  6 : Constant  Value=KTQD_SetSpdDeltaLongMPH_mph
  7 : Constant  Value=KTQD_CCActiveMetSpdHi_kph
  8 : Constant  Value=KTQD_CCActiveMetSpdHiMPH_mph
  AND1 : Logic  AllPortsSameDT=off  OutDataTypeStr=boolean
  CC Speed Setting Mode : Stateflow chart  TreatAsAtomicUnit=on
      settings: PortSchema="{\"entries\":[{\"content\":{\"sides\":[{\"content\":{\"connectorIds\":[\"In5\",\"In12\",\"In4\",\"In3\",\"In9\",\"In6\",\"In7\",\"In8\",\"In1\",\"In2\",\"In11\",\"In10\"]},\"type\":\"ConnectorPlacement.EquallySpacedRectSide\",\"uuid\":\"331c8dfa-4564-419d-9323-fdbf8561d50b\"},{\"content\":{\"connectorIds\":[\"Out1\",\"Out2\"],\"side\":\"RIGHT\"},\"type\":\"ConnectorPlacement.EquallySpacedRectSide\",\"uuid\":\"71cb1444-7708-4b6f-91dd-d8a1c8c14ea8\"},{\"content\":{\"connectorIds\":[],\"side\":\"TOP\"},\"type\":\"ConnectorPlacement.EquallySpacedRectSide\",\"uuid\":\"6ecf38bb-d171-491a-a8b2-073f135e7039\"}]},\"type\":\"ConnectorPlacement.EquallySpacedConnector\",\"uuid\":\"fc3afa97-6e6e-4933-9aff-7c8f8cbb1702\"}],\"packageUris\":[\"http://schema.mathworks.com/mf0/Connector/R2020b\"],\"version\":\"1.0\"}"
  Cast To Single : DataTypeConversion  OutDataTypeStr=int8
  Data Type Conversion : DataTypeConversion  OutDataTypeStr=uint8
  Data Type Conversion1 : DataTypeConversion  OutDataTypeStr=uint8
  ONE : Constant  Value=ONE_INT
  Product : Product
  Relational Operator2 : RelationalOperator  Operator===  OutDataTypeStr=boolean  RndMeth=Simplest
  Relational Operator4 : RelationalOperator  Operator===  OutDataTypeStr=boolean  RndMeth=Simplest
  Round : Rounding  Operator=round
  Specific_STATE_ChangeToSTANDBY : Stateflow chart  TreatAsAtomicUnit=on
  Switch{1..6} (6 alike) : Switch  Criteria=u2 ~= 0
      settings: AttributesFormatString=%<Criteria>
  standby : Constant  Value=ENUM_ADASCCSTA_STANDBY
  zero : Constant  Value=ZERO_INT
  zero1 : Constant  Value=KPH2MPH
  VTQD_CCSetSpd_kph : Outport
  VTQD_SWCCCSpdResetFinish_flg : Outport  Port=2
  wires:
  Data Type Conversion1/1 -> Switch5/1
  8/1 -> Switch6/3
  7/1 -> Switch5/3
  VINP_SmartEcoModeSW_flg/1 -> [VINP_SmartEcoModeSW_flg]
  5/1 -> Product/1
  zero1/1 -> Product/2
  Data Type Conversion/1 -> Switch6/1
  Product/1 -> Data Type Conversion/1
  Switch6/1 -> Switch2/1
  [VINP_SmartEcoModeSW_flg] -> Switch6/2
  3/1 -> Data Type Conversion1/1
  [VINP_SmartEcoModeSW_flg] -> Switch5/2
  [VINP_Distanceunit_flg] -> Switch2/2
  Switch5/1 -> Switch2/3
  CC Speed Setting Mode/1(VTQD_CCSetSpd_kph) -> Round/1
  Round/1 -> Cast To Single/1
  [VINP_Distanceunit_flg] -> CC Speed Setting Mode/6(VINP_Distanceunit_flg)
  6/1 -> Switch4/1
  4/1 -> Switch4/3
  [VINP_Distanceunit_flg] -> Switch4/2
  " 2"/1 -> Switch3/1
  " 1"/1 -> Switch3/3
  [VINP_Distanceunit_flg] -> Switch3/2
  VINP_Distanceunit_flg/1 -> [VINP_Distanceunit_flg]
  Relational Operator4/1 -> AND1/2
  Relational Operator2/1 -> AND1/1
  zero/1 -> Relational Operator4/2
  standby/1 -> Relational Operator2/2
  ONE/1 -> Switch1/1
  AND1/1 -> Switch1/2
  [VVMC_CCCtrlSta_enum] -> Relational Operator2/1
  Cast To Single/1 -> Switch1/3, Relational Operator4/1
  1/1 -> CC Speed Setting Mode/3(KTQD_SetSpdDeltaLongFit_kph)
  2/1 -> CC Speed Setting Mode/2(KTQD_SetSpdDeltaShort_kph)
  VVMC_CCCtrlSta_enum/1 -> [VVMC_CCCtrlSta_enum]
  [VVMC_CCCtrlSta_enum] -> Specific_STATE_ChangeToSTANDBY/1(VVMC_CCCtrlSta_enum)
  Specific_STATE_ChangeToSTANDBY/1(VTQD_CCChangeToSTANDBY_flg) -> [VTQD_ChangeToSTANDBY_flg]  "VTQD_CCChangeToSTANDBY_flg"
  [VTQD_ChangeToSTANDBY_flg] -> CC Speed Setting Mode/12(VTQD_ChangeToSTANDBY_flg)
  [VVMC_CCCtrlSta_enum] -> CC Speed Setting Mode/5(VVMC_CCCtrlSta_enum)
  VTQD_SetSpdDeltaLongFit_kph/1 -> [VTQD_SetSpdDeltaLongFit_kph]
  [VTQD_SetSpdDeltaLongFit_kph] -> CC Speed Setting Mode/4(VTQD_SetSpdDeltaLongFit_kph)
  VVMC_MeterIndSpeed_raw32/1 -> [VVMC_MeterIndSpeed_raw32]
  [VVMC_MeterIndSpeed_raw32] -> CC Speed Setting Mode/9(VVMC_MeterIndSpeed_raw32)
  Switch1/1 -> [VTQD_CCSetSpd_kph]
  [VTQD_CCSetSpd_kph] -> VTQD_CCSetSpd_kph/1
  CC Speed Setting Mode/2(VTQD_CCSpdResetFinish_flg) -> [VTQD_CCSpdResetFinish_flg]  "VTQD_SWCCCSpdResetFinish_flg"
  [VTQD_CCSpdResetFinish_flg] -> VTQD_SWCCCSpdResetFinish_flg/1
  "VTQD_SWCResUpPress_enum  "/1 -> [VTQD_SWCResUpPress_enum]
  [VTQD_SWCResUpPress_enum] -> CC Speed Setting Mode/11(VTQD_SWCResUpPress_enum)
  "VTQD_SWCSetDownPress_enum  "/1 -> [VTQD_SWCSetDownPress_enum]
  [VTQD_SWCSetDownPress_enum] -> CC Speed Setting Mode/10(VTQD_SWCSetDownPress_enum)
  Switch2/1 -> [KTQD_CCActiveMetSpdHi_raw32]
  [KTQD_CCActiveMetSpdHi_raw32] -> CC Speed Setting Mode/7(KTQD_CCActiveMetSpdHi_raw32)
  [KTQD_CCActiveMetSpdLo_raw32] -> CC Speed Setting Mode/8(KTQD_CCActiveMetSpdLo_raw32)
  Switch3/1 -> [KTQD_CCActiveMetSpdLo_raw32]
  Switch4/1 -> [KTQD_SetSpdDeltaLong_kph]
  [KTQD_SetSpdDeltaLong_kph] -> CC Speed Setting Mode/1(KTQD_SetSpdDeltaLong_kph)

== system tqdtqr_rebuild_V3/Input_Convert/Signal function/SWC1 SWC2 status/SWC_Subsystem/Speed Setting Mode/Else Speed Setting On ==
  In : Inport
  Action Port : ActionPort  ActionPortLabel=else
  Data Type Conversion : DataTypeConversion
  Out : Outport
  wires:
  In/1 -> Data Type Conversion/1
  Data Type Conversion/1 -> Out/1

== system tqdtqr_rebuild_V3/Input_Convert/Signal function/SWC1 SWC2 status/SWC_Subsystem/Speed Setting Mode/ISA Speed Setting ON ==
  VINP_ADASVehSpdLim_kph : Inport
  VINP_SmartEcoModeSW_flg : Inport  Port=2
  Action Port : ActionPort  ActionPortLabel=elseif( u4~= 0)
  8 : Constant  Value=KTQD_SmartEcoLimitSpd_kph
  Data Type Conversion : DataTypeConversion
  Min : MinMax  Inputs=2
  Switch : Switch  Criteria=u2 ~= 0
      settings: AttributesFormatString=%<Criteria>
  VTQD_ISASetSpd_kph : Outport
  wires:
  Data Type Conversion/1 -> VTQD_ISASetSpd_kph/1
  8/1 -> Min/1
  VINP_SmartEcoModeSW_flg/1 -> Switch/2
  VINP_ADASVehSpdLim_kph/1 -> Switch/3, Min/2
  Switch/1 -> Data Type Conversion/1
  Min/1 -> Switch/1

== system tqdtqr_rebuild_V3/Input_Convert/Signal function/SWC1 SWC2 status/SWC_Subsystem/Speed Setting Mode/MSA Speed Setting ON ==
  note: MSA SPEED SETTING MODE
  VVMC_MSACrlSta_enum : Inport
  "VTQD_SWCResUpPress_enum  " : Inport  Port=2
  "VTQD_SWCSetDownPress_enum  " : Inport  Port=3
  VVMC_MeterIndSpeed_raw32 : Inport  Port=4
  VTQD_SetSpdDeltaLongFit_kph : Inport  Port=5
  VINP_Distanceunit_flg : Inport  Port=6
  VINP_SmartEcoModeSW_flg : Inport  Port=7
  Action Port : ActionPort  InitializeStates=reset  ActionPortLabel=elseif( u3~= 0)
  " 1" : Constant  Value=KTQD_MSAActiveMetSpdLoMPH_mph
  " 80" : Constant  Value=KTQD_MSAActiveMetSpdLo_kph
  1 : Constant  Value=KTQD_SetSpdDeltaShort_kph
  160 : Constant  Value=KTQD_MSAActiveMetSpdHi_kph
  2 : Constant  Value=KTQD_SmartEcoLimitSpd_kph
  3 : Constant  Value=KTQD_SetSpdDeltaLongMPH_mph
  4 : Constant  Value=KTQD_SmartEcoLimitSpd_kph
  5 : Constant  Value=KTQD_SetSpdDeltaLong_kph
  6 : Constant  Value=KTQD_MSAActiveMetSpdHiMPH_mph
  AND1 : Logic  AllPortsSameDT=off  OutDataTypeStr=boolean
  Cast To Single : DataTypeConversion  OutDataTypeStr=int8
  Data Type Conversion : DataTypeConversion  OutDataTypeStr=uint8
  Data Type Conversion1 : DataTypeConversion  OutDataTypeStr=uint8
  Delta Long Fit Base : Constant  Value=KTQD_SetSpdDeltaLongFit_kph
  MSA : Stateflow chart  TreatAsAtomicUnit=on
      settings: PortSchema="{\"entries\":[{\"content\":{\"sides\":[{\"content\":{\"connectorIds\":[\"In9\",\"In6\",\"In5\",\"In4\",\"In7\",\"In8\",\"In1\",\"In2\",\"In12\",\"In10\",\"In11\",\"In3\"]},\"type\":\"ConnectorPlacement.EquallySpacedRectSide\",\"uuid\":\"4fee65fe-2e32-4dfc-9c8c-ef7087e97952\"},{\"content\":{\"connectorIds\":[\"Out1\"],\"side\":\"RIGHT\"},\"type\":\"ConnectorPlacement.EquallySpacedRectSide\",\"uuid\":\"8d915692-cb0b-4a06-a57e-690cea51e532\"},{\"content\":{\"connectorIds\":[],\"side\":\"TOP\"},\"type\":\"ConnectorPlacement.EquallySpacedRectSide\",\"uuid\":\"3fa43362-4ddf-4693-9d82-d4f790f00c9c\"}]},\"type\":\"ConnectorPlacement.EquallySpacedConnector\",\"uuid\":\"c1a6cfdc-58f2-45b0-af62-575976a00cf2\"}],\"packageUris\":[\"http://schema.mathworks.com/mf0/Connector/R2020b\"],\"version\":\"1.0\"}"
  ONE : Constant  Value=ONE_INT
  Product : Product
  Relational Operator2 : RelationalOperator  Operator===  OutDataTypeStr=boolean  RndMeth=Simplest
  Relational Operator4 : RelationalOperator  Operator===  OutDataTypeStr=boolean  RndMeth=Simplest
  Round : Rounding  Operator=round
  Specific_STATE_ChangeToOFF : Stateflow chart  TreatAsAtomicUnit=on
  Switch{1..6} (6 alike) : Switch  Criteria=u2 ~= 0
      settings: AttributesFormatString=%<Criteria>
  standby : Constant  Value=ENUM_ADASMSASTA_STANDBY
  zero : Constant  Value=ZERO_INT
  zero1 : Constant  Value=KPH2MPH
  VSCP_MSASetSpd_kph : Outport
  wires:
  Data Type Conversion1/1 -> Switch5/1
  6/1 -> Switch6/3
  160/1 -> Switch5/3
  Data Type Conversion/1 -> Switch6/1
  [VINP_SmartEcoModeSW_flg] -> Switch5/2
  [VINP_SmartEcoModeSW_flg] -> Switch6/2
  [VINP_Distanceunit_flg] -> Switch2/2
  2/1 -> Data Type Conversion1/1
  Product/1 -> Data Type Conversion/1
  Switch6/1 -> Switch2/1
  Switch5/1 -> Switch2/3
  zero1/1 -> Product/2
  4/1 -> Product/1
  VINP_SmartEcoModeSW_flg/1 -> [VINP_SmartEcoModeSW_flg]
  MSA/1(VTQD_MSASetSpd_kph) -> Round/1
  Round/1 -> Cast To Single/1
  [VINP_Distanceunit_flg] -> MSA/4(VINP_Distanceunit_flg)
  3/1 -> Switch4/1
  5/1 -> Switch4/3
  [VINP_Distanceunit_flg] -> Switch4/2
  " 1"/1 -> Switch3/1
  " 80"/1 -> Switch3/3
  [VINP_Distanceunit_flg] -> Switch3/2
  VINP_Distanceunit_flg/1 -> [VINP_Distanceunit_flg]
  Relational Operator4/1 -> AND1/2
  [VINP_MSACrlSta_enum] -> Relational Operator2/1
  Relational Operator2/1 -> AND1/1
  Cast To Single/1 -> Switch1/3, Relational Operator4/1
  ONE/1 -> Switch1/1
  standby/1 -> Relational Operator2/2
  zero/1 -> Relational Operator4/2
  AND1/1 -> Switch1/2
  [VINP_MSACrlSta_enum] -> Specific_STATE_ChangeToOFF/1(VINP_MSACrlSta_enum)
  Specific_STATE_ChangeToOFF/1(VTQD_ChangeToOFF_flg) -> [VTQD_ChangeToOFF_flg]  "VTQD_ChangeToOFF_flg"
  [VTQD_ChangeToOFF_flg] -> MSA/5(VTQD_ChangeToOFF_flg)
  1/1 -> MSA/2(KTQD_SetSpdDeltaShort_kph)
  VVMC_MSACrlSta_enum/1 -> [VINP_MSACrlSta_enum]
  Delta Long Fit Base/1 -> MSA/11(KTQD_SetSpdDeltaLongFit_kph)
  [VINP_MSACrlSta_enum] -> MSA/9(VVMC_MSACrlSta_enum)
  VVMC_MeterIndSpeed_raw32/1 -> [VVMC_MeterIndSpeed_raw32]
  [VVMC_MeterIndSpeed_raw32] -> MSA/6(VVMC_MeterIndSpeed_raw32)
  "VTQD_SWCResUpPress_enum  "/1 -> [VTQD_SWCResUpPress_enum]
  [VTQD_SWCResUpPress_enum] -> MSA/12(VTQD_SWCResUpPress_enum)
  VTQD_SetSpdDeltaLongFit_kph/1 -> [VTQD_SetSpdDeltaLongFit_kph]
  [VTQD_SetSpdDeltaLongFit_kph] -> MSA/10(VTQD_SetSpdDeltaLongFit_kph)
  "VTQD_SWCSetDownPress_enum  "/1 -> [VTQD_SWCSetDownPress_enum]
  [VTQD_SWCSetDownPress_enum] -> MSA/3(VTQD_SWCSetDownPress_enum)
  Switch1/1 -> [VSCP_MSASetSpd_kph]
  [VSCP_MSASetSpd_kph] -> VSCP_MSASetSpd_kph/1
  Switch2/1 -> [KTQD_MSAActiveMetSpdHi_raw32]
  [KTQD_MSAActiveMetSpdHi_raw32] -> MSA/7(KTQD_MSAActiveMetSpdHi_raw32)
  Switch3/1 -> [KTQD_MSAActiveMetSpdLo_raw32]
  [KTQD_MSAActiveMetSpdLo_raw32] -> MSA/8(KTQD_MSAActiveMetSpdLo_raw32)
  Switch4/1 -> [KTQD_SetSpdDeltaLong_kph]
  [KTQD_SetSpdDeltaLong_kph] -> MSA/1(KTQD_SetSpdDeltaLong_kph)

== system tqdtqr_rebuild_V3/Input_Convert/Signal function/SWC1 SWC2 status/SWC_Subsystem/Speed Setting Mode/VTQD_SWCResUpPress_enum ==
  note: Long press or Short press
  INPUT : Inport
  task_time_s : Inport  Port=2
  AND : Logic  AllPortsSameDT=off  OutDataTypeStr=boolean
  AND1 : Logic  AllPortsSameDT=off  OutDataTypeStr=boolean
  Constant2 : Constant  Value=KTQD_SetSpdShortPLim_s
  Constant3 : Constant  Value=KTQD_SetSpdLongPLim_s
  Constant4 : Constant  Value=ENUM_SWCBOTTONPRESS_LONGPRESS
  Constant5 : Constant  Value=ENUM_SWCBOTTONPRESS_SHORTPRESS
  Constant6 : Constant  Value=ENUM_SWCBOTTONPRESS_NOPRESS
  Delay : Delay  DelayLength=1  InitialCondition=boolean(0)
      settings: AttributesFormatString=%<InitialCondition>
  DelayEnable_LONG_PRESS1 : hcu_lib/Basic_Blocks/DelayEnable
  DelayEnable_SHORT_PRESS1 : hcu_lib/Basic_Blocks/DelayEnable
  Detect Decrease : simulink/Logic and Bit Operations/Detect Decrease  vinit=boolean(0)  OutDataTypeStr=boolean
  Detect Decrease4 : simulink/Logic and Bit Operations/Detect Decrease  vinit=boolean(0)  OutDataTypeStr=boolean
  NOT : Logic  Operator=NOT  AllPortsSameDT=off  OutDataTypeStr=boolean
  NOT1 : Logic  Operator=NOT  AllPortsSameDT=off  OutDataTypeStr=boolean
  SR_Latch : hcu_lib/Basic_Blocks/SR_Latch
  Switch : Switch  Criteria=u2 ~= 0
      settings: AttributesFormatString=%<Criteria>
  Switch3 : Switch  Criteria=u2 ~= 0
      settings: AttributesFormatString=%<Criteria>
  OUTPUT : Outport
  wires:
  Switch/1 -> OUTPUT/1
  Constant6/1 -> Switch3/3
  Constant4/1 -> Switch/1
  Constant5/1 -> Switch3/1
  [Long_press_falling_edge] -> Switch/2
  Detect Decrease4/1 -> [Short_press_falling_Edge]
  [task_time_s] -> DelayEnable_LONG_PRESS1/3
  [task_time_s] -> DelayEnable_SHORT_PRESS1/3
  Constant2/1 -> DelayEnable_SHORT_PRESS1/2
  Constant3/1 -> DelayEnable_LONG_PRESS1/2
  DelayEnable_SHORT_PRESS1/1 -> Detect Decrease4/1
  Switch3/1 -> Switch/3
  DelayEnable_LONG_PRESS1/1 -> [Long_press_falling_edge]
  task_time_s/1 -> [task_time_s]
  INPUT/1 -> [INPUT]
  [Long_press_falling_edge] -> Delay/1
  Delay/1 -> NOT/1
  NOT/1 -> AND/2
  AND/1 -> DelayEnable_LONG_PRESS1/1
  [INPUT] -> AND/1
  [Long_press_falling_edge] -> SR_Latch/1
  AND1/1 -> DelayEnable_SHORT_PRESS1/1
  [INPUT] -> AND1/1
  SR_Latch/1 -> NOT1/1
  NOT1/1 -> AND1/2
  [INPUT] -> Detect Decrease/1
  Detect Decrease/1 -> SR_Latch/2
  [Short_press_falling_Edge] -> Switch3/2

== system tqdtqr_rebuild_V3/Input_Convert/Signal function/SWC1 SWC2 status/SWC_Subsystem/Speed Setting Mode/VTQD_SWCSetDownPress_enum ==
  note: Long press or Short press
  INPUT : Inport
  task_time_s : Inport  Port=2
  AND : Logic  AllPortsSameDT=off  OutDataTypeStr=boolean
  AND1 : Logic  AllPortsSameDT=off  OutDataTypeStr=boolean
  Constant1 : Constant  Value=ENUM_SWCBOTTONPRESS_LONGPRESS
  Constant2 : Constant  Value=KTQD_SetSpdShortPLim_s
  Constant3 : Constant  Value=KTQD_SetSpdLongPLim_s
  Constant7 : Constant  Value=ENUM_SWCBOTTONPRESS_SHORTPRESS
  Constant8 : Constant  Value=ENUM_SWCBOTTONPRESS_NOPRESS
  Delay : Delay  DelayLength=1  InitialCondition=boolean(0)
      settings: AttributesFormatString=%<InitialCondition>
  DelayEnable_LONG_PRESS1 : hcu_lib/Basic_Blocks/DelayEnable
  DelayEnable_SHORT_PRESS1 : hcu_lib/Basic_Blocks/DelayEnable
  Detect Decrease : simulink/Logic and Bit Operations/Detect Decrease  vinit=boolean(0)  OutDataTypeStr=boolean
  Detect Decrease4 : simulink/Logic and Bit Operations/Detect Decrease  vinit=boolean(0)  OutDataTypeStr=boolean
  NOT : Logic  Operator=NOT  AllPortsSameDT=off  OutDataTypeStr=boolean
  NOT1 : Logic  Operator=NOT  AllPortsSameDT=off  OutDataTypeStr=boolean
  SR_Latch : hcu_lib/Basic_Blocks/SR_Latch
  Switch : Switch  Criteria=u2 ~= 0
      settings: AttributesFormatString=%<Criteria>
  Switch3 : Switch  Criteria=u2 ~= 0
      settings: AttributesFormatString=%<Criteria>
  OUTPUT : Outport
  wires:
  Switch/1 -> OUTPUT/1
  Constant8/1 -> Switch3/3
  Constant1/1 -> Switch/1
  Constant7/1 -> Switch3/1
  [Long_press_falling_edge] -> Switch/2
  Detect Decrease4/1 -> [Short_press_falling_Edge]
  [task_time_s] -> DelayEnable_LONG_PRESS1/3
  [task_time_s] -> DelayEnable_SHORT_PRESS1/3
  Constant2/1 -> DelayEnable_SHORT_PRESS1/2
  Constant3/1 -> DelayEnable_LONG_PRESS1/2
  DelayEnable_SHORT_PRESS1/1 -> Detect Decrease4/1
  Switch3/1 -> Switch/3
  DelayEnable_LONG_PRESS1/1 -> [Long_press_falling_edge]
  task_time_s/1 -> [task_time_s]
  INPUT/1 -> [INPUT]
  [Long_press_falling_edge] -> Delay/1
  Delay/1 -> NOT/1
  NOT/1 -> AND/2
  AND/1 -> DelayEnable_LONG_PRESS1/1
  [INPUT] -> AND/1
  [Long_press_falling_edge] -> SR_Latch/1
  AND1/1 -> DelayEnable_SHORT_PRESS1/1
  [INPUT] -> AND1/1
  SR_Latch/1 -> NOT1/1
  NOT1/1 -> AND1/2
  [INPUT] -> Detect Decrease/1
  Detect Decrease/1 -> SR_Latch/2
  [Short_press_falling_Edge] -> Switch3/2
